simulink model "arq_select_rep_p5_2006b"  (Simulink 6.5)
settings: Solver=VariableStepDiscrete  StartTime=0.0  StopTime=50  MaxStep=inf  RelTol=1e-3
PostLoadFcn:
  | arq_selective_repeat_settings;
undefined symbols (not defined in the file or in its folder): des_figposition, des_subsystemblock, des_subsysteminport, des_subsystemoutport, des_subsystemsupportblock
libraries: simeventsserver1 x7, simeventssink1 x7, simeventsattributes1 x6, simeventstranslate1 x6, simeventsgates1 x4, simeventsrouting1 x4, simeventsgenerators1 x3, simeventsprobes1 x2, simulink x2, simeventsqueue1 x2, simeventsinfo x1
CloseFcn:
  | clear Pe;
  | clear SWS;
  | clear Tframe;
  | clear Tprop;
settings Model: Creator=jbryan  LastModifiedBy=pablopad  ExtModeAutoUpdateStatusClock=off
settings DebuggingCC: MultiTaskDSMMsg=warning  MultiTaskCondExecSysMsg=none
settings RTWCC: IncludeERTFirstTime=on
settings SimEventsCC: propLogEventsScheduled=0  propLogEventsExecuted=0  propLogDepartureEvents=0  propDisplayEventCalendar=0

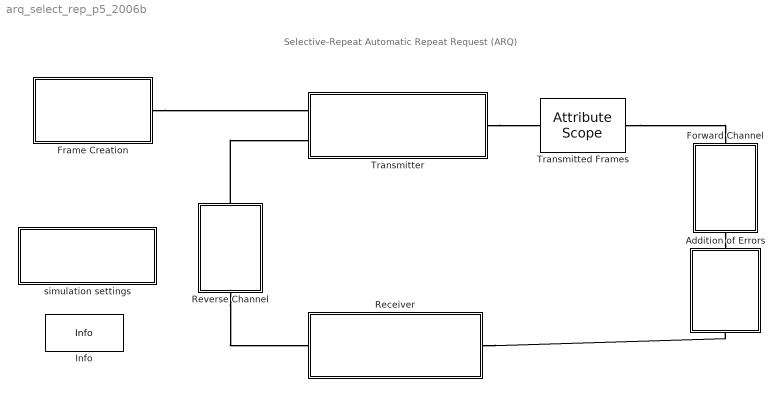
== system arq_select_rep_p5_2006b ==
  note: Selective-Repeat Automatic Repeat Request (ARQ)
  Addition of Errors : Subsystem  Orientation=down
  Forward Channel : Subsystem  Orientation=down
  Frame Creation : Subsystem
  Info : simeventsinfo/Info  SystemSampleTime=-1
  Receiver : Subsystem  Orientation=left
  Reverse Channel : Subsystem  Orientation=up
  Transmitted Frames : simeventssink1/Attribute Scope  Priority=1  SystemSampleTime=-1  PlotType=Stem  InputType=Attribute  NumInputs=1  AttributeNameY=seqNum  XInputOptionSignal=Event time  XInputOptionEntity=Event time  AttributeNameX=Count  EnableEntityOutport=on  XMin=0  XMax=51  XLimitExceededOption=Stretch axis limits  YLimitExceededOption=Stretch axis limits  AxisGrid=on  AxisLegend=off  LineDisables=""  LineColors=b  LineStyles=-  LineMarkers=.  OpenScopeAtSimStart=on  Title=Transmitted Frames  YLabel=Frame Number  XLabel=Time  FigurePosition=des_figposition([46 18 22 25])  AxisZoom=off  DataStoreOption=Limited  DataPointsLimit=10000  StatNumberArrived=Off  ShowCountPlotted=off  ShowToolbar=off
      settings: YMin=0  YMax=60
  Transmitter : Subsystem
  simulation settings : Subsystem  mask(simulation settings){SWS=7, Tframe=.1, Tprop=1, Pe=.15}
      mask prompts: SWS "Sliding window size:"; Tframe "Time to transmit frame:"; Tprop "Propagation time:"; Pe "Probability of erroneous frame:"
      mask help:
      | Parameter settings for Selective Repeat Automatic Repeat Request (ARQ) model.
      |
      | Sliding window size: Maximum number of unacknowledged frames allowed in transit at any time
      |
      | Time to transmit frame: Amount of time it takes transmitter to send out all bits in a given frame
      |
      | Propagation time: Amount of time for a frame to propagate one way from the transmitter to the receiver or vice versa.  This should be longer than the time to transmit a frame.
      |
      | Probability of erroneous frame: Probability that a frame will be corrupted in transit, requiring it to be resent
      mask init:
      | arq_select_rep_p5_settings;
      mask Help: eval('simeventsdemohelp')
      mask Display: disp('Double-click to change\nsimulation settings')
  connections:
  Transmitter/RConn1 -- Transmitted Frames/LConn1
  Forward Channel/RConn1 -- Addition of Errors/LConn1
  Receiver/LConn1 -- Addition of Errors/RConn1
  Frame Creation/RConn1 -- Transmitter/LConn1
  Reverse Channel/LConn1 -- Receiver/RConn1
  Reverse Channel/RConn1 -- Transmitter/LConn2
  Transmitted Frames/RConn1 -- Forward Channel/LConn1

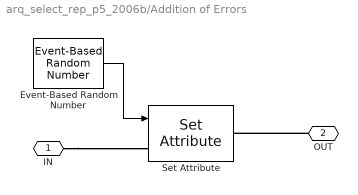
== system arq_select_rep_p5_2006b/Addition of Errors ==
  Event-Based Random Number : simeventsgenerators1/Signal Generators/Event-Based Random Number  SystemSampleTime=-1  distribution=Bernoulli  meanExp=1  minUnif=0  maxUnif=1  pOneBern=Pe  pSuccessBino=0.5  numTrialBino=1  meanNorm=0  stdNorm=1  minTri=1  maxTri=3  modeTri=2  thresholdLogn=0  scaleLogn=1  shapeLogn=1  pSuccessGeo=0.5  meanPoiss=1  thresholdLogl=0  scaleLogl=1  thresholdGam=0  scaleGam=1  shapeGam=1  minBeta=0  maxBeta=1  shape1Beta=1  shape2Beta=1  minUnid=0  maxUnid=1  numValueUnid=2  thresholdWbl=0  scaleWbl=1  shapeWbl=1  valueVecCont=[0 1]  cdfVecCont=[0 1]  valueVecDisc=[0 1]  probVecDisc=[0.5 0.5]  seed=12345  IsProcessed=on
  Set Attribute : simeventsattributes1/Set Attribute  Priority=1  SystemSampleTime=-1  Attribute1From=From signal port A1  Attribute1Name=crc_check  Attribute1DataType=Double  Attribute1Value=0  Attribute1Create=on  Attribute2From=Off  Attribute2Name=Attribute2  Attribute2DataType=Double  Attribute2Value=0  Attribute2Create=on  Attribute3From=Off  Attribute3Name=Attribute3  Attribute3DataType=Double  Attribute3Value=0  Attribute3Create=on  Attribute4From=Off  Attribute4Name=Attribute4  Attribute4DataType=Double  Attribute4Value=0  Attribute4Create=on  StatNumberDeparted=Off
  IN : PMIOPort  Port=1  Side=Left
  OUT : PMIOPort  Orientation=left  Port=2  Side=Right
  wires:
  Event-Based Random Number/1 -> Set Attribute/1
  connections:
  OUT/RConn1 -- Set Attribute/RConn1
  IN/RConn1 -- Set Attribute/LConn1

== system arq_select_rep_p5_2006b/Forward Channel ==
  Infinite Server : simeventsserver1/Infinite Server  Priority=1  SystemSampleTime=-1  ServiceTimeFrom=Dialog  ServiceTime=Tprop  AttributeName=ServiceTime  PriorityServiceCompletion=200  StatNumberDeparted=Off  StatNumberInBlock=Off  StatPendingEntity=Off  StatNumberPending=Off  StatAverageWait=Off
  IN : PMIOPort  Port=1  Side=Left
  OUT : PMIOPort  Orientation=left  Port=2  Side=Right
  connections:
  IN/RConn1 -- Infinite Server/LConn1
  Infinite Server/RConn1 -- OUT/RConn1

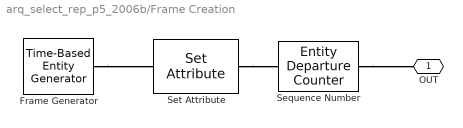
== system arq_select_rep_p5_2006b/Frame Creation ==
  Frame Generator : simeventsgenerators1/Entity Generators/Time-Based Entity Generator  Priority=1  DialogController=des_ddg_create  DialogControllerArgs=DataTag3  SystemSampleTime=-1  GenerateEntitiesUpon=Intergeneration time from dialog  Distribution=Exponential  Minimum=0  Maximum=3  Mean=1  InitialSeed=2367  Period=1  PriorityEntityGeneration=1000  GenerateEntityAtSimulationStart=on  ResponseWhenBlocked=Pause generation  ResponseWhenUnblocked=Immediate restart  EntityType=Blank  StatNumberDeparted=Off  StatPendingEntity=Off  StatAverageIntergenerationTime=Off
  Sequence Number : simeventsprobes1/Entity Departure Counter  Priority=1  SystemSampleTime=-1  NumberDepartedToSignal=Off  NumberDepartedToAttribute=On  NumberDepartedAttributeName=seqNum  CounterResetTypeOption=Off  CounterResetEdgeOption=Rising  SpecifyEventPriority=off  PriorityEntityCounterReset=1
  Set Attribute : simeventsattributes1/Set Attribute  Priority=1  SystemSampleTime=-1  Attribute1From=Specify via dialog  Attribute1Name=seqNum  Attribute1DataType=Double  Attribute1Value=0  Attribute1Create=on  Attribute2From=Off  Attribute2Name=Attribute2  Attribute2DataType=Double  Attribute2Value=0  Attribute2Create=on  Attribute3From=Off  Attribute3Name=Attribute3  Attribute3DataType=Double  Attribute3Value=0  Attribute3Create=on  Attribute4From=Off  Attribute4Name=Attribute4  Attribute4DataType=Double  Attribute4Value=0  Attribute4Create=on  StatNumberDeparted=Off
  OUT : PMIOPort  Orientation=left  Port=1  Side=Right
  connections:
  Sequence Number/RConn1 -- OUT/RConn1
  Frame Generator/RConn1 -- Set Attribute/LConn1
  Set Attribute/RConn1 -- Sequence Number/LConn1

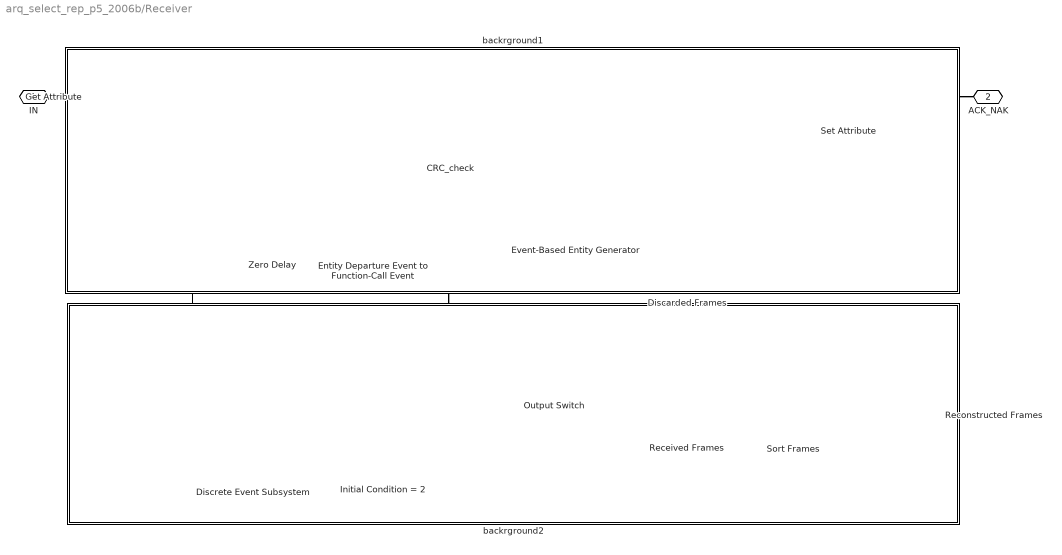
== system arq_select_rep_p5_2006b/Receiver ==
  CRC_check : simeventssink1/Signal Scope  Priority=1  SystemSampleTime=-1  PlotType=Stair  InputType=Signal  NumInputs=1  AttributeNameY=Count  XInputOptionSignal=Event time  XInputOptionEntity=Event time  AttributeNameX=Count  EnableEntityOutport=on  XMin=0  XMax=51  XLimitExceededOption=Stretch axis limits  YLimitExceededOption=Stretch axis limits  AxisGrid=on  AxisLegend=off  LineDisables=""  LineColors=b  LineStyles=-  LineMarkers=.  OpenScopeAtSimStart=on  Title=CRC Check  YLabel=""  XLabel=Time  FigurePosition=des_figposition([24 18 22 25])  AxisZoom=off  DataStoreOption=Limited  DataPointsLimit=10000  StatNumberArrived=Off  ShowCountPlotted=off  ShowToolbar=off
      settings: YMin=0  YMax=1.1
  Discarded Frames : simeventssink1/Attribute Scope  Priority=1  SystemSampleTime=-1  PlotType=Stair  InputType=Attribute  NumInputs=1  AttributeNameY=seqNum  XInputOptionSignal=Event time  XInputOptionEntity=Event time  AttributeNameX=Count  EnableEntityOutport=off  XMin=0  XMax=40  XLimitExceededOption=Stretch axis limits  YLimitExceededOption=Stretch axis limits  AxisGrid=on  AxisLegend=off  LineDisables=""  LineColors=b  LineStyles=-  LineMarkers=.  OpenScopeAtSimStart=on  Title=Discarded Frames  YLabel=Sequence Number  XLabel=Time  FigurePosition=des_figposition([2 18 22 25])  AxisZoom=off  DataStoreOption=Limited  DataPointsLimit=10000  StatNumberArrived=Off  ShowCountPlotted=off  ShowToolbar=off
      settings: YMin=0  YMax=40
  Discrete Event Subsystem : Subsystem  LoadFcn=des_subsystemblock(gcb, 'load');  InitFcn=des_subsystemblock(gcb, 'init');  StartFcn=des_subsystemblock(gcb, 'start');  StopFcn=des_subsystemblock(gcb, 'stop');
      settings: CopyFcn=des_subsystemblock(gcb, 'copy');  DeleteFcn=des_subsystemblock(gcb, 'delete');  UndoDeleteFcn=des_subsystemblock(gcb, 'undodelete');  ModelCloseFcn=des_subsystemblock(gcb, 'modelclose');  PreSaveFcn=des_subsystemblock(gcb, 'presave');  NameChangeFcn=des_subsystemblock(gcb, 'namechange');  OpenFcn=des_subsystemblock(gcb, 'open');  ParentCloseFcn=des_subsystemblock(gcb, 'parentclose');
      mask Type: Discrete Event Subsystem
      mask Help: helpview(simeventsbhelp);
  Entity Departure Event to Function-Call Event : simeventstranslate1/Entity Departure Event to Function-Call Event  Priority=1  SystemSampleTime=-1  TimingFunctionCallF1=After entity departure  EnableE1Port=off  EnableF2Port=off  TimingFunctionCallF2=Before entity departure  EnableE2Port=off  StatNumberDeparted=Off  StatNumberF1Calls=Off  StatNumberF2Calls=Off
  Event-Based Entity Generator : simeventsgenerators1/Entity Generators/Event-Based Entity Generator  Priority=1  DialogController=des_ddg_create  DialogControllerArgs=DataTag17  SystemSampleTime=-1  GenerateEntitiesUpon=Function call from port fcn  SignalEdgeType=Rising  SpecifyEventPriority=on  PriorityEntityGeneration=1  GenerateEntityAtSimulationStart=off  AllowBlocking=off  ResponseDuringBlockage=Discard generated entities  EntityType=Blank  StatNumberDeparted=Off  StatPendingEntity=Off  StatAverageIntergenerationTime=Off
  Get Attribute : simeventsattributes1/Get Attribute  Priority=1  SystemSampleTime=-1  Attribute1To=On  Attribute1Name=crc_check  Attribute1Missing=Error  Attribute1DefaultValue=0  Attribute2To=Off  Attribute2Name=Attribute2  Attribute2Missing=Error  Attribute2DefaultValue=0  Attribute3To=Off  Attribute3Name=Attribute3  Attribute3Missing=Error  Attribute3DefaultValue=0  Attribute4To=Off  Attribute4Name=Attribute4  Attribute4Missing=Error  Attribute4DefaultValue=0  StatNumberDeparted=Off
  Initial Condition = 2 : simeventsgates1/Signal Latch  Priority=1  SystemSampleTime=-1  InitialMemoryValue=2  WriteMemoryUpon=Sample time hit from port wts  MemoryWriteEdgeOption=Rising  SpecifyWriteEventPriority=on  PriorityMemoryWrite=1  ReadMemoryUpon=Write to memory event  MemoryReadEdgeOption=Falling  SpecifyReadEventPriority=on  PriorityMemoryRead=7000  ReportMemoryState=off  ReportMemoryUponWrite=on  ReportMemoryUponRead=off
  Output Switch : simeventsrouting1/Output Switch  Priority=1  SystemSampleTime=-1  NumberOutputPorts=2  SwitchingCriterion=From signal port p  InitialSeed=34567  AttributeName=crc_check  SpecifyEventPriority=off  PriorityOutputSwitchSelectPort=100  StatNumberDeparted=Off  StatLastDeparturePort=Off
  Received Frames : simeventssink1/Attribute Scope  Priority=1  SystemSampleTime=-1  PlotType=Stair  InputType=Attribute  NumInputs=1  AttributeNameY=seqNum  XInputOptionSignal=Event time  XInputOptionEntity=Event time  AttributeNameX=Count  EnableEntityOutport=on  XMin=0  XMax=51  XLimitExceededOption=Stretch axis limits  YLimitExceededOption=Stretch axis limits  AxisGrid=on  AxisLegend=off  LineDisables=""  LineColors=b  LineStyles=-  LineMarkers=.  OpenScopeAtSimStart=on  Title=Received Frames  YLabel=Frame Number  XLabel=Time  FigurePosition=des_figposition([68 18 22 25])  AxisZoom=off  DataStoreOption=Limited  DataPointsLimit=10000  StatNumberArrived=Off  ShowCountPlotted=off  ShowToolbar=off
      settings: YMin=0  YMax=60
  Reconstructed Frames : simeventssink1/Attribute Scope  Priority=1  SystemSampleTime=-1  PlotType=Stair  InputType=Attribute  NumInputs=1  AttributeNameY=seqNum  XInputOptionSignal=Event time  XInputOptionEntity=Event time  AttributeNameX=Count  EnableEntityOutport=off  XMin=0  XMax=51  XLimitExceededOption=Stretch axis limits  YLimitExceededOption=Stretch axis limits  AxisGrid=on  AxisLegend=off  LineDisables=""  LineColors=b  LineStyles=-  LineMarkers=.  OpenScopeAtSimStart=on  Title=Reconstructed Frames  YLabel=Sequence Number  XLabel=Time  FigurePosition=des_figposition([68 45 22 25])  AxisZoom=off  DataStoreOption=Limited  DataPointsLimit=10000  StatNumberArrived=Off  ShowCountPlotted=off  ShowToolbar=off
      settings: YMin=0  YMax=60
  Set Attribute : simeventsattributes1/Set Attribute  Priority=1  SystemSampleTime=-1  Attribute1From=From signal port A1  Attribute1Name=ack  Attribute1DataType=Double  Attribute1Value=0  Attribute1Create=on  Attribute2From=Off  Attribute2Name=Attribute2  Attribute2DataType=Double  Attribute2Value=0  Attribute2Create=on  Attribute3From=Off  Attribute3Name=Attribute3  Attribute3DataType=Double  Attribute3Value=0  Attribute3Create=on  Attribute4From=Off  Attribute4Name=Attribute4  Attribute4DataType=Double  Attribute4Value=0  Attribute4Create=on  StatNumberDeparted=Off
  Sort Frames : Subsystem
  Zero Delay : simeventsserver1/Infinite Server  Priority=1  SystemSampleTime=-1  ServiceTimeFrom=Dialog  ServiceTime=0  AttributeName=ServiceTime  PriorityServiceCompletion=10  StatNumberDeparted=Off  StatNumberInBlock=Off  StatPendingEntity=Off  StatNumberPending=Off  StatAverageWait=Off
  backrground1 : Subsystem
      mask Display: disp('')
  backrground2 : Subsystem
      mask Display: disp('')
  IN : PMIOPort  Port=1  Side=Left
  ACK_NAK : PMIOPort  Orientation=left  Port=2  Side=Right
  wires:
  Get Attribute/1 -> Discrete Event Subsystem/1(Din), Set Attribute/1, CRC_check/1
  Entity Departure Event to Function-Call Event/1 -> Event-Based Entity Generator/1
  Discrete Event Subsystem/1(Dout) -> Initial Condition = 2/1, Initial Condition = 2/2
  Initial Condition = 2/1 -> Output Switch/1
  connections:
  Set Attribute/RConn1 -- ACK_NAK/RConn1
  IN/RConn1 -- Get Attribute/LConn1
  Get Attribute/RConn1 -- Zero Delay/LConn1
  Entity Departure Event to Function-Call Event/LConn1 -- Zero Delay/RConn1
  Event-Based Entity Generator/RConn1 -- Set Attribute/LConn1
  Entity Departure Event to Function-Call Event/RConn1 -- Output Switch/LConn1
  Received Frames/RConn1 -- Sort Frames/LConn1
  Sort Frames/RConn1 -- Reconstructed Frames/LConn1
  Discarded Frames/LConn1 -- Output Switch/RConn1
  Received Frames/LConn1 -- Output Switch/RConn2

== system arq_select_rep_p5_2006b/Reverse Channel ==
  Infinite Server : simeventsserver1/Infinite Server  Priority=1  SystemSampleTime=-1  ServiceTimeFrom=Dialog  ServiceTime=Tprop  AttributeName=ServiceTime  PriorityServiceCompletion=300  StatNumberDeparted=Off  StatNumberInBlock=Off  StatPendingEntity=Off  StatNumberPending=Off  StatAverageWait=Off
  IN : PMIOPort  Port=1  Side=Left
  OUT : PMIOPort  Orientation=left  Port=2  Side=Right
  connections:
  Infinite Server/RConn1 -- OUT/RConn1
  IN/RConn1 -- Infinite Server/LConn1

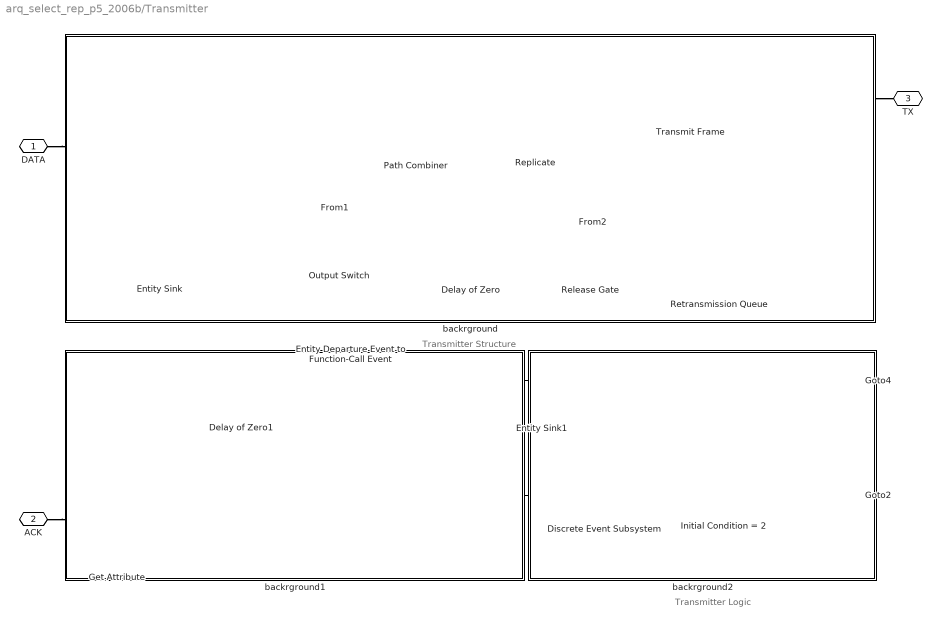
== system arq_select_rep_p5_2006b/Transmitter ==
  note: Transmitter Structure
  note: Transmitter Logic
  Delay of Zero : simeventsserver1/Infinite Server  Orientation=left  Priority=1  SystemSampleTime=-1  ServiceTimeFrom=Dialog  ServiceTime=0  AttributeName=ServiceTime  PriorityServiceCompletion=10  StatNumberDeparted=Off  StatNumberInBlock=Off  StatPendingEntity=Off  StatNumberPending=Off  StatAverageWait=Off
  Delay of Zero1 : simeventsserver1/Infinite Server  Priority=1  SystemSampleTime=-1  ServiceTimeFrom=Dialog  ServiceTime=0  AttributeName=ServiceTime  PriorityServiceCompletion=10  StatNumberDeparted=Off  StatNumberInBlock=Off  StatPendingEntity=Off  StatNumberPending=Off  StatAverageWait=Off
  Discrete Event Subsystem : Subsystem  LoadFcn=des_subsystemblock(gcb, 'load');  InitFcn=des_subsystemblock(gcb, 'init');  StartFcn=des_subsystemblock(gcb, 'start');  StopFcn=des_subsystemblock(gcb, 'stop');
      settings: CopyFcn=des_subsystemblock(gcb, 'copy');  DeleteFcn=des_subsystemblock(gcb, 'delete');  UndoDeleteFcn=des_subsystemblock(gcb, 'undodelete');  ModelCloseFcn=des_subsystemblock(gcb, 'modelclose');  PreSaveFcn=des_subsystemblock(gcb, 'presave');  NameChangeFcn=des_subsystemblock(gcb, 'namechange');  OpenFcn=des_subsystemblock(gcb, 'open');  ParentCloseFcn=des_subsystemblock(gcb, 'parentclose');
      mask Type: Discrete Event Subsystem
      mask Help: helpview(simeventsbhelp);
  Entity Departure Event to Function-Call Event : simeventstranslate1/Entity Departure Event to Function-Call Event  Priority=1  SystemSampleTime=-1  TimingFunctionCallF1=After entity departure  EnableE1Port=off  EnableF2Port=off  TimingFunctionCallF2=Before entity departure  EnableE2Port=off  StatNumberDeparted=Off  StatNumberF1Calls=Off  StatNumberF2Calls=Off
  Entity Sink : simeventssink1/Entity Sink  Orientation=left  Priority=1  SystemSampleTime=-1  AvailableForArrivals=on  StatNumberArrived=Off
  Entity Sink1 : simeventssink1/Entity Sink  Priority=1  SystemSampleTime=-1  AvailableForArrivals=on  StatNumberArrived=Off
  Get Attribute : simeventsattributes1/Get Attribute  Priority=1  SystemSampleTime=-1  Attribute1To=On  Attribute1Name=ack  Attribute1Missing=Error  Attribute1DefaultValue=0  Attribute2To=Off  Attribute2Name=seqNum  Attribute2Missing=Error  Attribute2DefaultValue=0  Attribute3To=Off  Attribute3Name=Attribute3  Attribute3Missing=Error  Attribute3DefaultValue=0  Attribute4To=Off  Attribute4Name=Attribute4  Attribute4Missing=Error  Attribute4DefaultValue=0  StatNumberDeparted=Off
  Initial Condition = 2 : simeventsgates1/Signal Latch  Priority=1  SystemSampleTime=-1  InitialMemoryValue=2  WriteMemoryUpon=Sample time hit from port wts  MemoryWriteEdgeOption=Rising  SpecifyWriteEventPriority=on  PriorityMemoryWrite=1  ReadMemoryUpon=Write to memory event  MemoryReadEdgeOption=Falling  SpecifyReadEventPriority=on  PriorityMemoryRead=7000  ReportMemoryState=off  ReportMemoryUponWrite=on  ReportMemoryUponRead=off
  Output Switch : simeventsrouting1/Output Switch  Orientation=left  Priority=1  SystemSampleTime=-1  NumberOutputPorts=2  SwitchingCriterion=From signal port p  InitialSeed=34567  AttributeName=Attribute1  SpecifyEventPriority=off  PriorityOutputSwitchSelectPort=2  StatNumberDeparted=Off  StatLastDeparturePort=Off
  Path Combiner : simeventsrouting1/Path Combiner  Priority=1  SystemSampleTime=-1  NumberInputPorts=2  InputPortPrecedence=IN1 port  InitialSeed=45675  SpecifyEventPriority=off  PriorityPathCombinerPortPrecedenceSelection=4100  StatNumberDeparted=Off  StatLastArrivalPort=Off
  Release Gate : simeventsgates1/Release Gate  Orientation=left  Priority=1  SystemSampleTime=-1  OpenGateUpon=Function call from port fcn  SignalEdgeOption=Rising  SpecifyEventPriority=on  PriorityGateRelease=2  StatNumberDeparted=Off
  Replicate : simeventsrouting1/Replicate  Priority=1  SystemSampleTime=-1  NumberOutputPorts=2  ReplicateEntityWhen=All entity output ports are not blocked  OutputPortPrecedence=OUT1 port  InitialSeed=56789  ActionUponBlocking=Discard entity  StatNumberArrived=Off  StatNumberDeparted=Off
  Retransmission Queue : simeventsqueue1/FIFO Queue  Orientation=left  Priority=1  SystemSampleTime=-1  Capacity=SWS  StatNumberDeparted=Off  StatNumberInBlock=Off  StatPendingEntity=Off  StatAverageWait=Off  StatAverageQueueLength=Off
  Transmit Frame : simeventsserver1/Single Server  Priority=1  SystemSampleTime=-1  ServiceTimeFrom=Dialog  ServiceTime=Tframe  AttributeName=ServiceTime  PriorityServiceCompletion=100  PermitPreemption=off  SortingAttributeName=PriorityAttributeName  SortingDirection=Ascending  WriteToAttribute=off  ResidualAttributeName=ResidualServiceTime  CreateAttribute=on  StatNumberDeparted=Off  StatNumberInBlock=Off  StatNumberPreempted=Off  StatPendingEntity=Off  StatAverageWait=Off  StatUtilization=Off
  backrground : Subsystem
      mask Display: disp('')
  backrground1 : Subsystem
      mask Display: disp('')
  backrground2 : Subsystem
      mask Display: disp('')
  DATA : PMIOPort  Port=1  Side=Left
  ACK : PMIOPort  Port=2  Side=Left
  TX : PMIOPort  Orientation=left  Port=3  Side=Right
  wires:
  [p] -> Output Switch/1
  [retx] -> Release Gate/1
  Entity Departure Event to Function-Call Event/1 -> [retx]
  Get Attribute/1 -> Discrete Event Subsystem/1(Din)
  Initial Condition = 2/1 -> [p]
  Discrete Event Subsystem/1(Dout) -> Initial Condition = 2/1, Initial Condition = 2/2
  connections:
  Delay of Zero1/RConn1 -- Entity Departure Event to Function-Call Event/LConn1
  Entity Departure Event to Function-Call Event/RConn1 -- Entity Sink1/LConn1
  ACK/RConn1 -- Get Attribute/LConn1
  Get Attribute/RConn1 -- Delay of Zero1/LConn1
  Path Combiner/RConn1 -- Replicate/LConn1
  Retransmission Queue/RConn1 -- Release Gate/LConn1
  Delay of Zero/LConn1 -- Release Gate/RConn1
  Replicate/RConn2 -- Retransmission Queue/LConn1
  Replicate/RConn1 -- Transmit Frame/LConn1
  Output Switch/LConn1 -- Delay of Zero/RConn1
  Transmit Frame/RConn1 -- TX/RConn1
  DATA/RConn1 -- Path Combiner/LConn2
  Output Switch/RConn1 -- Path Combiner/LConn1
  Entity Sink/LConn1 -- Output Switch/RConn2

== system arq_select_rep_p5_2006b/simulation settings ==

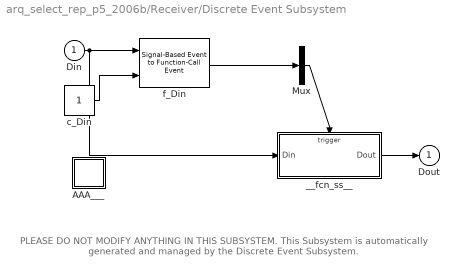
== system arq_select_rep_p5_2006b/Receiver/Discrete Event Subsystem ==
  note: PLEASE DO NOT MODIFY ANYTHING IN THIS SUBSYSTEM.
      | This Subsystem is automatically generated and
      | managed by the Discrete Event Subsystem.
  Din : Inport  PortDimensions=1  DataType=double
  AAA___ : Subsystem  LoadFcn=des_subsystemsupportblock(gcb, 'load');  InitFcn=des_subsystemsupportblock(gcb, 'init');  StartFcn=des_subsystemsupportblock(gcb, 'start');  StopFcn=des_subsystemsupportblock(gcb, 'stop');
      settings: CopyFcn=des_subsystemsupportblock(gcb, 'copy');  DeleteFcn=des_subsystemsupportblock(gcb, 'delete');  UndoDeleteFcn=des_subsystemsupportblock(gcb, 'undodelete');  ModelCloseFcn=des_subsystemsupportblock(gcb, 'modelclose');  PreSaveFcn=des_subsystemsupportblock(gcb, 'presave');  NameChangeFcn=des_subsystemsupportblock(gcb, 'namechange');  OpenFcn=des_subsystemsupportblock(gcb, 'open');  ParentCloseFcn=des_subsystemsupportblock(gcb, 'parentclose');
  Mux : Mux  Inputs=1
  __fcn_ss__ : Subsystem  TreatAsAtomicUnit=on
      settings: PropExecContextOutsideSubsystem=on
  c_Din : Constant  Value=1  OutDataType=sfix(16)  ConRadixGroup=Use specified scaling  OutScaling=2^0  SampleTime=inf  FramePeriod=inf
  f_Din : simeventstranslate1/Signal-Based Event to Function-Call Event  Priority=1  SystemSampleTime=-1  GenerateFunctionCallUpon=Sample time hit from port ts  SignalEdgeOption=Rising  EnableE1Port=on  EnableF2Port=off  EnableE2Port=off  SpecifyEventPriority=on  PriorityFunctionCall=1  FunctionCallDelayFrom=Dialog  DelayFunctionCall=0  StatNumberF1Calls=Off  StatNumberF2Calls=Off
  Dout : Outport
  wires:
  __fcn_ss__/1(Dout) -> Dout/1
  f_Din/1 -> Mux/1
  c_Din/1 -> f_Din/2
  Mux/1 -> __fcn_ss__/Trigger
  Din/1 -> f_Din/1, __fcn_ss__/1(Din)

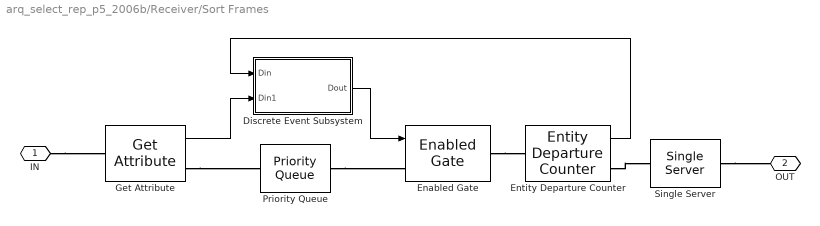
== system arq_select_rep_p5_2006b/Receiver/Sort Frames ==
  Discrete Event Subsystem : Subsystem  LoadFcn=des_subsystemblock(gcb, 'load');  InitFcn=des_subsystemblock(gcb, 'init');  StartFcn=des_subsystemblock(gcb, 'start');  StopFcn=des_subsystemblock(gcb, 'stop');
      settings: CopyFcn=des_subsystemblock(gcb, 'copy');  DeleteFcn=des_subsystemblock(gcb, 'delete');  UndoDeleteFcn=des_subsystemblock(gcb, 'undodelete');  ModelCloseFcn=des_subsystemblock(gcb, 'modelclose');  PreSaveFcn=des_subsystemblock(gcb, 'presave');  NameChangeFcn=des_subsystemblock(gcb, 'namechange');  OpenFcn=des_subsystemblock(gcb, 'open');  ParentCloseFcn=des_subsystemblock(gcb, 'parentclose');
      mask Type: Discrete Event Subsystem
      mask Help: helpview(simeventsbhelp);
  Enabled Gate : simeventsgates1/Enabled Gate  Priority=1  SystemSampleTime=-1  SpecifyEventPriority=off  PriorityGateEnableOpenClose=2000  StatNumberDeparted=Off
  Entity Departure Counter : simeventsprobes1/Entity Departure Counter  Priority=1  SystemSampleTime=-1  NumberDepartedToSignal=On  NumberDepartedToAttribute=Off  NumberDepartedAttributeName=Count  CounterResetTypeOption=Off  CounterResetEdgeOption=Rising  SpecifyEventPriority=off  PriorityEntityCounterReset=1
  Get Attribute : simeventsattributes1/Get Attribute  Priority=1  SystemSampleTime=-1  Attribute1To=On  Attribute1Name=seqNum  Attribute1Missing=Error  Attribute1DefaultValue=0  Attribute2To=Off  Attribute2Name=Attribute2  Attribute2Missing=Error  Attribute2DefaultValue=0  Attribute3To=Off  Attribute3Name=Attribute3  Attribute3Missing=Error  Attribute3DefaultValue=0  Attribute4To=Off  Attribute4Name=Attribute4  Attribute4Missing=Error  Attribute4DefaultValue=0  StatNumberDeparted=Off
  Priority Queue : simeventsqueue1/Priority Queue  Priority=1  SystemSampleTime=-1  Capacity=inf  SortingAttributeName=seqNum  SortingDirection=Ascending  StatNumberDeparted=Off  StatNumberInBlock=Off  StatPendingEntity=Off  StatAverageWait=Off  StatAverageQueueLength=Off
  Single Server : simeventsserver1/Single Server  Priority=1  SystemSampleTime=-1  ServiceTimeFrom=Dialog  ServiceTime=0  AttributeName=ServiceTime  PriorityServiceCompletion=500  PermitPreemption=off  SortingAttributeName=PriorityAttributeName  SortingDirection=Ascending  WriteToAttribute=off  ResidualAttributeName=ResidualServiceTime  CreateAttribute=on  StatNumberDeparted=Off  StatNumberInBlock=Off  StatNumberPreempted=Off  StatPendingEntity=Off  StatAverageWait=Off  StatUtilization=Off
  IN : PMIOPort  Port=1  Side=Left
  OUT : PMIOPort  Orientation=left  Port=2  Side=Right
  wires:
  Get Attribute/1 -> Discrete Event Subsystem/2(Din1)
  Discrete Event Subsystem/1(Dout) -> Enabled Gate/1
  Entity Departure Counter/1 -> Discrete Event Subsystem/1(Din)
  connections:
  IN/RConn1 -- Get Attribute/LConn1
  Get Attribute/RConn1 -- Priority Queue/LConn1
  Priority Queue/RConn1 -- Enabled Gate/LConn1
  Enabled Gate/RConn1 -- Entity Departure Counter/LConn1
  Single Server/RConn1 -- OUT/RConn1
  Entity Departure Counter/RConn1 -- Single Server/LConn1

== system arq_select_rep_p5_2006b/Receiver/backrground1 ==

== system arq_select_rep_p5_2006b/Receiver/backrground2 ==

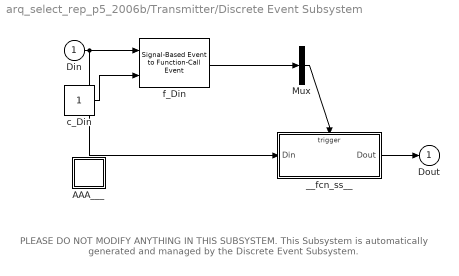
== system arq_select_rep_p5_2006b/Transmitter/Discrete Event Subsystem ==
  note: PLEASE DO NOT MODIFY ANYTHING IN THIS SUBSYSTEM.
      | This Subsystem is automatically generated and
      | managed by the Discrete Event Subsystem.
  Din : Inport  PortDimensions=1  DataType=double
  AAA___ : Subsystem  LoadFcn=des_subsystemsupportblock(gcb, 'load');  InitFcn=des_subsystemsupportblock(gcb, 'init');  StartFcn=des_subsystemsupportblock(gcb, 'start');  StopFcn=des_subsystemsupportblock(gcb, 'stop');
      settings: CopyFcn=des_subsystemsupportblock(gcb, 'copy');  DeleteFcn=des_subsystemsupportblock(gcb, 'delete');  UndoDeleteFcn=des_subsystemsupportblock(gcb, 'undodelete');  ModelCloseFcn=des_subsystemsupportblock(gcb, 'modelclose');  PreSaveFcn=des_subsystemsupportblock(gcb, 'presave');  NameChangeFcn=des_subsystemsupportblock(gcb, 'namechange');  OpenFcn=des_subsystemsupportblock(gcb, 'open');  ParentCloseFcn=des_subsystemsupportblock(gcb, 'parentclose');
  Mux : Mux  Inputs=1
  __fcn_ss__ : Subsystem  TreatAsAtomicUnit=on
      settings: PropExecContextOutsideSubsystem=on
  c_Din : Constant  Value=1  OutDataType=sfix(16)  ConRadixGroup=Use specified scaling  OutScaling=2^0  SampleTime=inf  FramePeriod=inf
  f_Din : simeventstranslate1/Signal-Based Event to Function-Call Event  Priority=1  SystemSampleTime=-1  GenerateFunctionCallUpon=Sample time hit from port ts  SignalEdgeOption=Rising  EnableE1Port=on  EnableF2Port=off  EnableE2Port=off  SpecifyEventPriority=on  PriorityFunctionCall=1  FunctionCallDelayFrom=Dialog  DelayFunctionCall=0  StatNumberF1Calls=Off  StatNumberF2Calls=Off
  Dout : Outport
  wires:
  __fcn_ss__/1(Dout) -> Dout/1
  f_Din/1 -> Mux/1
  c_Din/1 -> f_Din/2
  Mux/1 -> __fcn_ss__/Trigger
  Din/1 -> f_Din/1, __fcn_ss__/1(Din)

== system arq_select_rep_p5_2006b/Transmitter/backrground ==

== system arq_select_rep_p5_2006b/Transmitter/backrground1 ==

== system arq_select_rep_p5_2006b/Transmitter/backrground2 ==

== system arq_select_rep_p5_2006b/Receiver/Discrete Event Subsystem/AAA___ ==

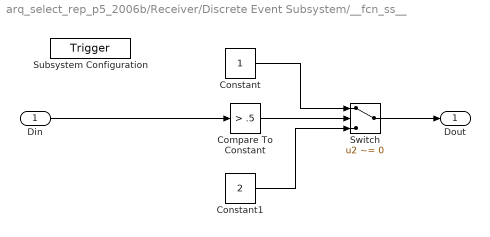
== system arq_select_rep_p5_2006b/Receiver/Discrete Event Subsystem/__fcn_ss__ ==
  Din : Inport  LoadFcn=des_subsysteminport(gcb, 'load');  InitFcn=des_subsysteminport(gcb, 'init');  StartFcn=des_subsysteminport(gcb, 'start');  StopFcn=des_subsysteminport(gcb, 'stop');  mask(Discrete Event Inport){PermitSubsystemEvents=on, TypeOfEvent=Sample time hit, SignalEdgeOption=Rising, SpecifyEventPriority=on, PrioritySubsystemEvent=1}
      mask prompts: PermitSubsystemEvents "Execute subsystem upon signal-based events"; TypeOfEvent "Type of signal-based event:"; SignalEdgeOption "Type of change in signal value:"; SpecifyEventPriority "Specify event priority for executing subsystem"; PrioritySubsystemEvent "Subsystem execution event priority:"
      mask help: Input port for a Discrete Event Subsystem block. This block can conditionally execute the subsystem upon signal-based events that meet specified criteria.
      mask init:
      | des_subsystemmask(gcb, 'init','apply')
      settings: CopyFcn=des_subsysteminport(gcb, 'copy');  DeleteFcn=des_subsysteminport(gcb, 'delete');  UndoDeleteFcn=des_subsysteminport(gcb, 'undodelete');  ModelCloseFcn=des_subsysteminport(gcb, 'modelclose');  PreSaveFcn=des_subsysteminport(gcb, 'presave');  NameChangeFcn=des_subsysteminport(gcb, 'namechange');  ParentCloseFcn=des_subsysteminport(gcb, 'parentclose');
      mask Help: helpview(simeventsbhelp);
      mask StyleString: checkbox,popup(Change in signal|Trigger|Sample time hit),popup(Rising|Falling|Either),checkbox,edit
      mask CallbackString: des_subsystemmask(gcb, 'cbPermitSubsystemEvents', 'noapply');|des_subsystemmask(gcb,'cbTypeOfEvent','noapply');||des_subsystemmask(gcb, 'cbSpecifyEventPriority', 'noapply');|
  Subsystem Configuration : TriggerPort  TriggerType=function-call
      settings: CopyFcn=des_subsystemconfigblock(gcb, 'copy');  DeleteFcn=des_subsystemconfigblock(gcb, 'delete');  UndoDeleteFcn=des_subsystemconfigblock(gcb, 'undodelete');
      mask Type: Subsystem Configuration
      mask Description: Configuration for a Discrete Event Subsystem block. Every discrete event subsystem window must contain exactly one copy of this configuration block. Do not delete this block.
      mask Help: helpview(simeventsbhelp);
      mask Display: disp('Do Not Delete');
  Compare To Constant : simulink/Logic and Bit Operations/Compare To Constant  SystemSampleTime=-1  relop=>  const=.5  LogicOutDataTypeMode=boolean  ZeroCross=off
  Constant : Constant  Value=1  OutDataType=sfix(16)  ConRadixGroup=Use specified scaling  OutScaling=2^0  SampleTime=inf  FramePeriod=inf
  Constant1 : Constant  Value=2  OutDataType=sfix(16)  ConRadixGroup=Use specified scaling  OutScaling=2^0  SampleTime=inf  FramePeriod=inf
  Switch : Switch  Criteria=u2 ~= 0
  Dout : Outport  LoadFcn=des_subsystemoutport(gcb, 'load');  InitFcn=des_subsystemoutport(gcb, 'init');  StartFcn=des_subsystemoutport(gcb, 'start');  StopFcn=des_subsystemoutport(gcb, 'stop');
      settings: CopyFcn=des_subsystemoutport(gcb, 'copy');  DeleteFcn=des_subsystemoutport(gcb, 'delete');  UndoDeleteFcn=des_subsystemoutport(gcb, 'undodelete');  ModelCloseFcn=des_subsystemoutport(gcb, 'modelclose');  PreSaveFcn=des_subsystemoutport(gcb, 'presave');  NameChangeFcn=des_subsystemoutport(gcb, 'namechange');  ParentCloseFcn=des_subsystemoutport(gcb, 'parentclose');
      mask Type: Discrete Event Outport
      mask Description: Provide an output port for a Discrete Event Subsystem block.
      mask Help: helpview(simeventsbhelp);
  wires:
  Din/1 -> Compare To Constant/1
  Compare To Constant/1 -> Switch/2
  Constant/1 -> Switch/1
  Constant1/1 -> Switch/3
  Switch/1 -> Dout/1

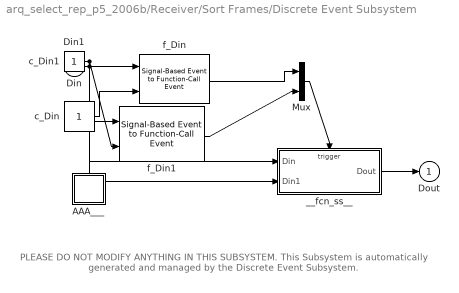
== system arq_select_rep_p5_2006b/Receiver/Sort Frames/Discrete Event Subsystem ==
  note: PLEASE DO NOT MODIFY ANYTHING IN THIS SUBSYSTEM.
      | This Subsystem is automatically generated and
      | managed by the Discrete Event Subsystem.
  Din : Inport  PortDimensions=1  DataType=double
  Din1 : Inport  Port=2  PortDimensions=1  DataType=double
  AAA___ : Subsystem  LoadFcn=des_subsystemsupportblock(gcb, 'load');  InitFcn=des_subsystemsupportblock(gcb, 'init');  StartFcn=des_subsystemsupportblock(gcb, 'start');  StopFcn=des_subsystemsupportblock(gcb, 'stop');
      settings: CopyFcn=des_subsystemsupportblock(gcb, 'copy');  DeleteFcn=des_subsystemsupportblock(gcb, 'delete');  UndoDeleteFcn=des_subsystemsupportblock(gcb, 'undodelete');  ModelCloseFcn=des_subsystemsupportblock(gcb, 'modelclose');  PreSaveFcn=des_subsystemsupportblock(gcb, 'presave');  NameChangeFcn=des_subsystemsupportblock(gcb, 'namechange');  OpenFcn=des_subsystemsupportblock(gcb, 'open');  ParentCloseFcn=des_subsystemsupportblock(gcb, 'parentclose');
  Mux : Mux  Inputs=2
  __fcn_ss__ : Subsystem  TreatAsAtomicUnit=on
      settings: PropExecContextOutsideSubsystem=on
  c_Din : Constant  Value=1  OutDataType=sfix(16)  ConRadixGroup=Use specified scaling  OutScaling=2^0  SampleTime=inf  FramePeriod=inf
  c_Din1 : Constant  Value=1  OutDataType=sfix(16)  ConRadixGroup=Use specified scaling  OutScaling=2^0  SampleTime=inf  FramePeriod=inf
  f_Din : simeventstranslate1/Signal-Based Event to Function-Call Event  Priority=1  SystemSampleTime=-1  GenerateFunctionCallUpon=Sample time hit from port ts  SignalEdgeOption=Rising  EnableE1Port=on  EnableF2Port=off  EnableE2Port=off  SpecifyEventPriority=off  PriorityFunctionCall=20  FunctionCallDelayFrom=Dialog  DelayFunctionCall=0  StatNumberF1Calls=Off  StatNumberF2Calls=Off
  f_Din1 : simeventstranslate1/Signal-Based Event to Function-Call Event  Priority=1  SystemSampleTime=-1  GenerateFunctionCallUpon=Sample time hit from port ts  SignalEdgeOption=Rising  EnableE1Port=on  EnableF2Port=off  EnableE2Port=off  SpecifyEventPriority=off  PriorityFunctionCall=20  FunctionCallDelayFrom=Dialog  DelayFunctionCall=0  StatNumberF1Calls=Off  StatNumberF2Calls=Off
  Dout : Outport
  wires:
  __fcn_ss__/1(Dout) -> Dout/1
  f_Din/1 -> Mux/1
  c_Din/1 -> f_Din/2
  Mux/1 -> __fcn_ss__/Trigger
  f_Din1/1 -> Mux/2
  c_Din1/1 -> f_Din1/2
  Din/1 -> f_Din/1, __fcn_ss__/1(Din)
  Din1/1 -> f_Din1/1, __fcn_ss__/2(Din1)

== system arq_select_rep_p5_2006b/Transmitter/Discrete Event Subsystem/AAA___ ==

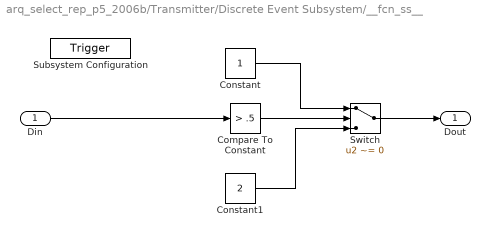
== system arq_select_rep_p5_2006b/Transmitter/Discrete Event Subsystem/__fcn_ss__ ==
  Din : Inport  LoadFcn=des_subsysteminport(gcb, 'load');  InitFcn=des_subsysteminport(gcb, 'init');  StartFcn=des_subsysteminport(gcb, 'start');  StopFcn=des_subsysteminport(gcb, 'stop');  mask(Discrete Event Inport){PermitSubsystemEvents=on, TypeOfEvent=Sample time hit, SignalEdgeOption=Rising, SpecifyEventPriority=on, PrioritySubsystemEvent=1}
      mask prompts: PermitSubsystemEvents "Execute subsystem upon signal-based events"; TypeOfEvent "Type of signal-based event:"; SignalEdgeOption "Type of change in signal value:"; SpecifyEventPriority "Specify event priority for executing subsystem"; PrioritySubsystemEvent "Subsystem execution event priority:"
      mask help: Input port for a Discrete Event Subsystem block. This block can conditionally execute the subsystem upon signal-based events that meet specified criteria.
      mask init:
      | des_subsystemmask(gcb, 'init','apply')
      settings: CopyFcn=des_subsysteminport(gcb, 'copy');  DeleteFcn=des_subsysteminport(gcb, 'delete');  UndoDeleteFcn=des_subsysteminport(gcb, 'undodelete');  ModelCloseFcn=des_subsysteminport(gcb, 'modelclose');  PreSaveFcn=des_subsysteminport(gcb, 'presave');  NameChangeFcn=des_subsysteminport(gcb, 'namechange');  ParentCloseFcn=des_subsysteminport(gcb, 'parentclose');
      mask Help: helpview(simeventsbhelp);
      mask StyleString: checkbox,popup(Change in signal|Trigger|Sample time hit),popup(Rising|Falling|Either),checkbox,edit
      mask CallbackString: des_subsystemmask(gcb, 'cbPermitSubsystemEvents', 'noapply');|des_subsystemmask(gcb,'cbTypeOfEvent','noapply');||des_subsystemmask(gcb, 'cbSpecifyEventPriority', 'noapply');|
  Subsystem Configuration : TriggerPort  TriggerType=function-call
      settings: CopyFcn=des_subsystemconfigblock(gcb, 'copy');  DeleteFcn=des_subsystemconfigblock(gcb, 'delete');  UndoDeleteFcn=des_subsystemconfigblock(gcb, 'undodelete');
      mask Type: Subsystem Configuration
      mask Description: Configuration for a Discrete Event Subsystem block. Every discrete event subsystem window must contain exactly one copy of this configuration block. Do not delete this block.
      mask Help: helpview(simeventsbhelp);
      mask Display: disp('Do Not Delete');
  Compare To Constant : simulink/Logic and Bit Operations/Compare To Constant  SystemSampleTime=-1  relop=>  const=.5  LogicOutDataTypeMode=boolean  ZeroCross=off
  Constant : Constant  Value=1  OutDataType=sfix(16)  ConRadixGroup=Use specified scaling  OutScaling=2^0  SampleTime=inf  FramePeriod=inf
  Constant1 : Constant  Value=2  OutDataType=sfix(16)  ConRadixGroup=Use specified scaling  OutScaling=2^0  SampleTime=inf  FramePeriod=inf
  Switch : Switch  Criteria=u2 ~= 0
  Dout : Outport  LoadFcn=des_subsystemoutport(gcb, 'load');  InitFcn=des_subsystemoutport(gcb, 'init');  StartFcn=des_subsystemoutport(gcb, 'start');  StopFcn=des_subsystemoutport(gcb, 'stop');
      settings: CopyFcn=des_subsystemoutport(gcb, 'copy');  DeleteFcn=des_subsystemoutport(gcb, 'delete');  UndoDeleteFcn=des_subsystemoutport(gcb, 'undodelete');  ModelCloseFcn=des_subsystemoutport(gcb, 'modelclose');  PreSaveFcn=des_subsystemoutport(gcb, 'presave');  NameChangeFcn=des_subsystemoutport(gcb, 'namechange');  ParentCloseFcn=des_subsystemoutport(gcb, 'parentclose');
      mask Type: Discrete Event Outport
      mask Description: Provide an output port for a Discrete Event Subsystem block.
      mask Help: helpview(simeventsbhelp);
  wires:
  Din/1 -> Compare To Constant/1
  Compare To Constant/1 -> Switch/2
  Constant/1 -> Switch/1
  Constant1/1 -> Switch/3
  Switch/1 -> Dout/1

== system arq_select_rep_p5_2006b/Receiver/Sort Frames/Discrete Event Subsystem/AAA___ ==

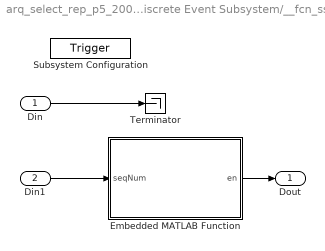
== system arq_select_rep_p5_2006b/Receiver/Sort Frames/Discrete Event Subsystem/__fcn_ss__ ==
  Din : Inport  LoadFcn=des_subsysteminport(gcb, 'load');  InitFcn=des_subsysteminport(gcb, 'init');  StartFcn=des_subsysteminport(gcb, 'start');  StopFcn=des_subsysteminport(gcb, 'stop');  mask(Discrete Event Inport){PermitSubsystemEvents=on, TypeOfEvent=Sample time hit, SignalEdgeOption=Rising, SpecifyEventPriority=off, PrioritySubsystemEvent=20}
      mask prompts: PermitSubsystemEvents "Execute subsystem upon signal-based events"; TypeOfEvent "Type of signal-based event:"; SignalEdgeOption "Type of change in signal value:"; SpecifyEventPriority "Specify event priority for executing subsystem"; PrioritySubsystemEvent "Subsystem execution event priority:"
      mask help: Input port for a Discrete Event Subsystem block. This block can conditionally execute the subsystem upon signal-based events that meet specified criteria.
      mask init:
      | des_subsystemmask(gcb, 'init','apply')
      settings: CopyFcn=des_subsysteminport(gcb, 'copy');  DeleteFcn=des_subsysteminport(gcb, 'delete');  UndoDeleteFcn=des_subsysteminport(gcb, 'undodelete');  ModelCloseFcn=des_subsysteminport(gcb, 'modelclose');  PreSaveFcn=des_subsysteminport(gcb, 'presave');  NameChangeFcn=des_subsysteminport(gcb, 'namechange');  ParentCloseFcn=des_subsysteminport(gcb, 'parentclose');
      mask Help: helpview(simeventsbhelp);
      mask StyleString: checkbox,popup(Change in signal|Trigger|Sample time hit),popup(Rising|Falling|Either),checkbox,edit
      mask CallbackString: des_subsystemmask(gcb, 'cbPermitSubsystemEvents', 'noapply');|des_subsystemmask(gcb,'cbTypeOfEvent','noapply');||des_subsystemmask(gcb, 'cbSpecifyEventPriority', 'noapply');|
  Din1 : Inport  LoadFcn=des_subsysteminport(gcb, 'load');  InitFcn=des_subsysteminport(gcb, 'init');  StartFcn=des_subsysteminport(gcb, 'start');  StopFcn=des_subsysteminport(gcb, 'stop');  Port=2  mask(Discrete Event Inport){PermitSubsystemEvents=on, TypeOfEvent=Sample time hit, SignalEdgeOption=Rising, SpecifyEventPriority=off, PrioritySubsystemEvent=20}
      mask prompts: PermitSubsystemEvents "Execute subsystem upon signal-based events"; TypeOfEvent "Type of signal-based event:"; SignalEdgeOption "Type of change in signal value:"; SpecifyEventPriority "Specify event priority for executing subsystem"; PrioritySubsystemEvent "Subsystem execution event priority:"
      mask help: Input port for a Discrete Event Subsystem block. This block can conditionally execute the subsystem upon signal-based events that meet specified criteria.
      mask init:
      | des_subsystemmask(gcb, 'init','apply')
      settings: CopyFcn=des_subsysteminport(gcb, 'copy');  DeleteFcn=des_subsysteminport(gcb, 'delete');  UndoDeleteFcn=des_subsysteminport(gcb, 'undodelete');  ModelCloseFcn=des_subsysteminport(gcb, 'modelclose');  PreSaveFcn=des_subsysteminport(gcb, 'presave');  NameChangeFcn=des_subsysteminport(gcb, 'namechange');  ParentCloseFcn=des_subsysteminport(gcb, 'parentclose');
      mask Help: helpview(simeventsbhelp);
      mask StyleString: checkbox,popup(Change in signal|Trigger|Sample time hit),popup(Rising|Falling|Either),checkbox,edit
      mask CallbackString: des_subsystemmask(gcb, 'cbPermitSubsystemEvents', 'noapply');|des_subsystemmask(gcb,'cbTypeOfEvent','noapply');||des_subsystemmask(gcb, 'cbSpecifyEventPriority', 'noapply');|
  Subsystem Configuration : TriggerPort  TriggerType=function-call
      settings: CopyFcn=des_subsystemconfigblock(gcb, 'copy');  DeleteFcn=des_subsystemconfigblock(gcb, 'delete');  UndoDeleteFcn=des_subsystemconfigblock(gcb, 'undodelete');
      mask Type: Subsystem Configuration
      mask Description: Configuration for a Discrete Event Subsystem block. Every discrete event subsystem window must contain exactly one copy of this configuration block. Do not delete this block.
      mask Help: helpview(simeventsbhelp);
      mask Display: disp('Do Not Delete');
  Embedded MATLAB Function : Stateflow chart
  Terminator : Terminator
  Dout : Outport  LoadFcn=des_subsystemoutport(gcb, 'load');  InitFcn=des_subsystemoutport(gcb, 'init');  StartFcn=des_subsystemoutport(gcb, 'start');  StopFcn=des_subsystemoutport(gcb, 'stop');
      settings: CopyFcn=des_subsystemoutport(gcb, 'copy');  DeleteFcn=des_subsystemoutport(gcb, 'delete');  UndoDeleteFcn=des_subsystemoutport(gcb, 'undodelete');  ModelCloseFcn=des_subsystemoutport(gcb, 'modelclose');  PreSaveFcn=des_subsystemoutport(gcb, 'presave');  NameChangeFcn=des_subsystemoutport(gcb, 'namechange');  ParentCloseFcn=des_subsystemoutport(gcb, 'parentclose');
      mask Type: Discrete Event Outport
      mask Description: Provide an output port for a Discrete Event Subsystem block.
      mask Help: helpview(simeventsbhelp);
  wires:
  Din1/1 -> Embedded MATLAB Function/1(seqNum)
  Embedded MATLAB Function/1(en) -> Dout/1
  Din/1 -> Terminator/1

== matlab function Receiver/Sort Frames/Discrete Event Subsystem/__fcn_ss__/Embedded MATLAB Function ==
  data: seqNum input inherited; en output inherited
function en = fcn(seqNum)
% Use a circular buffer to store all received frames.  
% A 1 indicates  that the frame has been received.

persistent buffer nextSeqNum index

% Initialize buffer to be all zeros
if isempty(buffer)
    buffer = zeros(100,1);
    nextSeqNum = 1;
    index = 1;
end

% We have received a new frame, set appropriate buffer element to 1
if seqNum >= nextSeqNum
    buffer(mod(index+seqNum-nextSeqNum-1,100)+1) = 1;
end

% Release frames from the front of the buffer
if buffer(index) == 1
    en = 1;
    buffer(index) = 0;
    index = mod(index,100)+1;
    nextSeqNum = nextSeqNum + 1;
else
    en = 0;
end
